simulink model "three_phase_FW_RL_low"  (R2022b)
settings: Solver=ode3  StartTime=0.0  StopTime=00.1  FixedStep=1e-4  RelTol=1e-3
libraries: spsDiodeLib x6, spsACVoltageSourceLib x3, spsCurrentMeasurementLib x2, spsVoltageMeasurementLib x2, spsGroundLib x1, spsSeriesRLCBranchLib x1, spsThreePhaseVIMeasurementLib x1, sps_lib x1
settings Model: Creator=mroun  LastModifiedBy=mroun

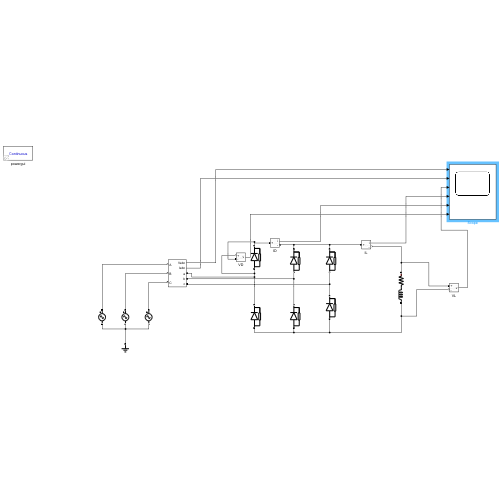
[thumbnail: Simulink's stored preview of the top-level diagram]
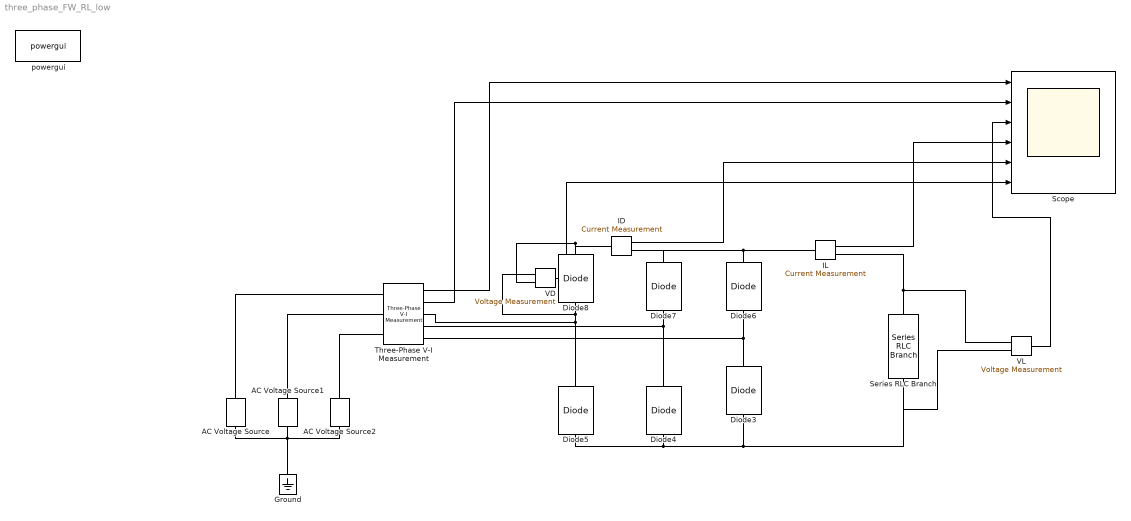
== system three_phase_FW_RL_low ==
  AC Voltage Source : spsACVoltageSourceLib/AC Voltage Source  Amplitude=400  Phase=0  Frequency=50  SampleTime=0  Measurements=None  BusType=swing  Pref=10e3  Qref=0  Qmin=-inf  Qmax=+inf
  AC Voltage Source1 : spsACVoltageSourceLib/AC Voltage Source  Amplitude=400  Phase=-120  Frequency=50  SampleTime=0  Measurements=None  BusType=swing  Pref=10e3  Qref=0  Qmin=-inf  Qmax=+inf
  AC Voltage Source2 : spsACVoltageSourceLib/AC Voltage Source  Amplitude=400  Phase=-240  Frequency=50  SampleTime=0  Measurements=None  BusType=swing  Pref=10e3  Qref=0  Qmin=-inf  Qmax=+inf
  Diode{3..8} (6 alike) : spsDiodeLib/Diode  Ron=0.001  Lon=0  Vf=0.8  IC=0  UseSnubber=0  Rs=500  Cs=250e-9  Measurements=off
  Ground : spsGroundLib/Ground  LConnTagsString=a
  ID : spsCurrentMeasurementLib/Current Measurement  PhasorSimulation=off  OutputType=Complex  PSBequivalent=0
  IL : spsCurrentMeasurementLib/Current Measurement  PhasorSimulation=off  OutputType=Complex  PSBequivalent=0
  Scope : Scope  NumInputPorts=6
  Series RLC Branch : spsSeriesRLCBranchLib/Series RLC Branch  LConnTagsString=__new0  RConnTagsString=__new0  BranchType=RL  Resistance=10  Inductance=.01  SetiL0=off  InitialCurrent=0  Capacitance=1e-6  Setx0=off  InitialVoltage=0  Measurements=None
  Three-Phase V-I Measurement : spsThreePhaseVIMeasurementLib/Three-Phase V-I Measurement  VoltageMeasurement=phase-to-ground  SetLabelV=off  LabelV=Vabc  Vpu=off  VpuLL=off  CurrentMeasurement=yes  SetLabelI=off  LabelI=Iabc  Ipu=off  Pbase=100e6  Vbase=500e3  OutputType=Complex  PhasorSimulation=off  PSBequivalent=0
  VD : spsVoltageMeasurementLib/Voltage Measurement  PhasorSimulation=off  OutputType=Complex  PSBequivalent=0
  VL : spsVoltageMeasurementLib/Voltage Measurement  PhasorSimulation=off  OutputType=Complex  PSBequivalent=0
  powergui : sps_lib/powergui  Priority=1  SimulationMode=Continuous  SampleTime=50e-6  frequency=60  Iterations=50  frequencyindice=50  Pbase=100e6  ErrMax=1e-4  UnitsV=kV  UnitsW=MW  buscounter=0  FunctionMessages=off  echomessages=off  EnableUseOfTLC=off  CurrentSourceSwitches=off  DisableSnubberDevices=off  DisableRonSwitches=off  DisableVfSwitches=off  DisplayEquations=off  AutomaticDiscreteSolvers=off  SolverType=Tustin/Backward Euler (TBE)  Interpol=off  ExternalGateDelay=off  methode=off  Ts=100  x0status=blocks  SPID=on  SwTol=0  HookPort=off  NonlinearTolerance=1e-4  nMaxIteration=100  ContinueOnMaxIteration=off  RestoreLinks=warning  ResistiveCurrentMeasurement=off  Frange=[0:2:500]  Ylog=off  Xlog=on  ShowGrid=off  save=off  variable=ZData  structure=0  ZoomFFT=off  StartTime=0.0  cycles=1  DisplayStyle=1  fundamental=60  FreqAxis=off  MaxFrequency=1000  frequencyindicesteady=1  RmsSteady=1  display=off
  wires:
  Three-Phase V-I Measurement/1 -> Scope/1
  Three-Phase V-I Measurement/2 -> Scope/2
  VL/1 -> Scope/3
  IL/1 -> Scope/4
  ID/1 -> Scope/5
  VD/1 -> Scope/6
  connections:
  AC Voltage Source2/LConn1 -- Ground/LConn1 -- AC Voltage Source1/LConn1 -- AC Voltage Source/LConn1
  AC Voltage Source2/RConn1 -- Three-Phase V-I Measurement/LConn3
  AC Voltage Source1/RConn1 -- Three-Phase V-I Measurement/LConn2
  AC Voltage Source/RConn1 -- Three-Phase V-I Measurement/LConn1
  Diode5/LConn1 -- VL/LConn2 -- Series RLC Branch/RConn1 -- Diode3/LConn1 -- Diode4/LConn1
  ID/RConn1 -- Diode7/RConn1 -- IL/LConn1 -- Diode6/RConn1
  Diode8/LConn1 -- VD/LConn1 -- Diode5/RConn1 -- Three-Phase V-I Measurement/RConn1
  Diode7/LConn1 -- Diode4/RConn1 -- Three-Phase V-I Measurement/RConn2
  Diode6/LConn1 -- Diode3/RConn1 -- Three-Phase V-I Measurement/RConn3
  VL/LConn1 -- IL/RConn1 -- Series RLC Branch/LConn1
  Diode8/RConn1 -- VD/LConn2 -- ID/LConn1
